simulink model "classifier"  (R2020b)
settings: Solver=FixedStepAuto  StartTime=0  StopTime=16  FixedStep=dt  RelTol=1e-3
values from neighbouring files (symbols this model uses):
  dt = 0.1    [create_data.m]    (also in run_classifier.m)
libraries: simulink x1
settings Model: Creator=alessandroantonucci  LastModifiedBy=alessandroantonucci
settings DataIOCC: LimitDataPoints=on  SaveOutput=off  SaveTime=off
settings OptimizationCC: BlockReduction=off  BooleanDataType=off  LifeSpan=inf
settings DebuggingCC: SaveWithParameterizedLinksMsg=none  UnderspecifiedInitializationDetection=Classic  MergeDetectMultiDrivingBlocksExec=none  SignalResolutionControl=TryResolveAllWithWarning  AllowSymbolicDim=off  SFUnexpectedBacktrackingDiag=warning  SFNoUnconditionalDefaultTransitionDiag=warning  SFExecutionAtInitializationDiag=none  ArithmeticOperatorsInVariantConditions=warning
settings HardwareCC: TargetUnknown=on
settings SFSimCC: SimUseLocalCustomCode=off  CustomCodeUndefinedFunction=UseInterfaceOnly  SimTargetLang=C++
settings RTWCC: RTWUseLocalCustomCode=off
settings CodeAppCC: StateflowObjectComments=on
settings GRTTargetCC: TargetLangStandard=C89/C90 (ANSI)

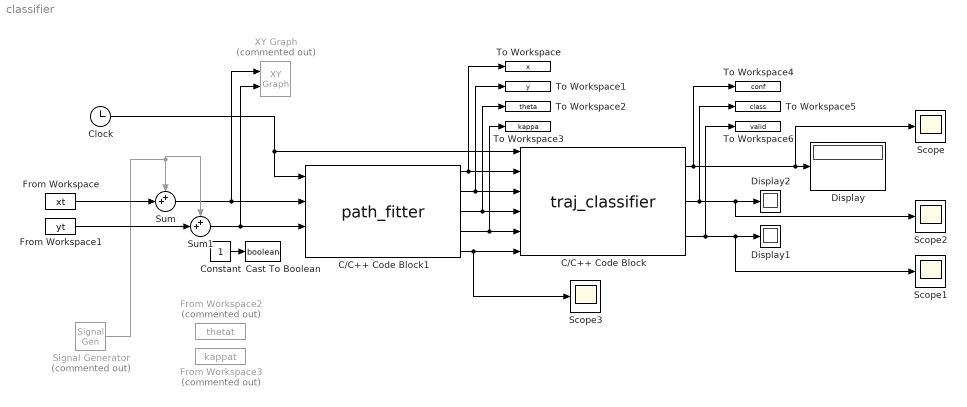
== system classifier ==
  C/C++ Code Block : S-Function  FunctionName=traj_classifier  SFunctionModules=traj_classifier_wrapper  SFunctionDeploymentMode=off  EnableBusSupport=off  mask(S-Function Builder){}
      mask help: Simulink:masks:SFunctionBuilder_MD
      mask init:
      | val = [[.9  0.75 0.75 1 1 .9 .9 1]',[1 1 0.75 0.75 .9 .9 1 .9]'];try , sys = get_param(gcb,'SfunBuilderFcnName');if isempty(sys), sys = get_param(gcb,'FunctionName'); end,catch, sys = get_param(gcb,'FunctionName'); end
      settings: CopyFcn=set_param(gcbh,'LinkStatus','none')  OpenFcn=sfunctionwizard(gcbh)
      mask Display:
      | plot(val(:,1),val(:,2))
      | disp(sys)
      | port_label('input',1,'time')
      | port_label('input',2,'in_x')
      | port_label('input',3,'in_y')
      | port_label('input',4,'in_theta')
      | port_label('input',5,'in_kappa')
      | port_label('input',6,'in_valid')
      | port_label('output',1,'out_conf')
      | port_label('output',2,'out_class')
      | port_label('output',3,'out_valid')
  C/C++ Code Block1 : S-Function  FunctionName=path_fitter  SFunctionModules=path_fitter_wrapper smooth  SFunctionDeploymentMode=off  EnableBusSupport=off  mask(S-Function Builder){}
      mask help: Simulink:masks:SFunctionBuilder_MD
      mask init: same as classifier/C/C++ Code Block
      settings: CopyFcn=set_param(gcbh,'LinkStatus','none')  OpenFcn=sfunctionwizard(gcbh)
      mask Display:
      | plot(val(:,1),val(:,2))
      | disp(sys)
      | port_label('input',1,'time')
      | port_label('input',2,'in_x')
      | port_label('input',3,'in_y')
      | port_label('input',4,'in_valid')
      | port_label('output',1,'out_x')
      | port_label('output',2,'out_y')
      | port_label('output',3,'out_theta')
      | port_label('output',4,'out_kappa')
      | port_label('output',5,'out_valid')
  Cast To Boolean : DataTypeConversion  OutDataTypeStr=boolean
  Clock : Clock
  Constant : Constant
  Display : Display
  Display1 : Display
  Display2 : Display
  From Workspace : FromWorkspace  VariableName=xt  SampleTime=dt
  From Workspace1 : FromWorkspace  VariableName=yt  SampleTime=dt
  From Workspace2 : FromWorkspace  Commented=on  VariableName=thetat  SampleTime=dt
  From Workspace3 : FromWorkspace  Commented=on  VariableName=kappat  SampleTime=dt
  Scope{,1..3} (4 alike) : Scope
  Signal Generator : SignalGenerator  Commented=on  WaveForm=random  Amplitude=0.1  Frequency=10
  Sum : Sum  Inputs=++|
  Sum1 : Sum  Inputs=++|
  To Workspace : ToWorkspace  VariableName=x  SaveFormat=Timeseries  SampleTime=-1
  To Workspace1 : ToWorkspace  VariableName=y  SaveFormat=Timeseries  SampleTime=-1
  To Workspace2 : ToWorkspace  VariableName=theta  SaveFormat=Timeseries  SampleTime=-1
  To Workspace3 : ToWorkspace  VariableName=kappa  SaveFormat=Timeseries  SampleTime=-1
  To Workspace4 : ToWorkspace  VariableName=conf  SaveFormat=Timeseries  SampleTime=-1
  To Workspace5 : ToWorkspace  VariableName=class  SaveFormat=Timeseries  SampleTime=-1
  To Workspace6 : ToWorkspace  VariableName=valid  SaveFormat=Timeseries  SampleTime=-1
  XY Graph : simulink/Sinks/XY Graph  Commented=on  xmin=0  xmax=15  ymin=0  ymax=15  st=-1
  wires:
  C/C++ Code Block/1 -> To Workspace4/1, Scope/1, Display/1
  Clock/1 -> C/C++ Code Block1/1, C/C++ Code Block/1
  Constant/1 -> Cast To Boolean/1
  C/C++ Code Block/2 -> To Workspace5/1, Scope2/1, Display2/1
  C/C++ Code Block/3 -> To Workspace6/1, Scope1/1, Display1/1
  Sum/1 -> XY Graph/1, C/C++ Code Block1/2
  Sum1/1 -> XY Graph/2, C/C++ Code Block1/3
  C/C++ Code Block1/4 -> C/C++ Code Block/5, To Workspace3/1
  C/C++ Code Block1/3 -> C/C++ Code Block/4, To Workspace2/1
  C/C++ Code Block1/2 -> C/C++ Code Block/3, To Workspace1/1
  C/C++ Code Block1/1 -> C/C++ Code Block/2, To Workspace/1
  Signal Generator/1 -> Sum1/1, Sum/1
  C/C++ Code Block1/5 -> Scope3/1, C/C++ Code Block/6
  From Workspace1/1 -> Sum1/2
  From Workspace/1 -> Sum/2
